simulink model "Q2_sim1"  (R2023b)
settings: Solver=VariableStepAuto  StartTime=0.0  StopTime=7  RelTol=1e-3
settings Model: Creator=avikd  LastModifiedBy=avikd

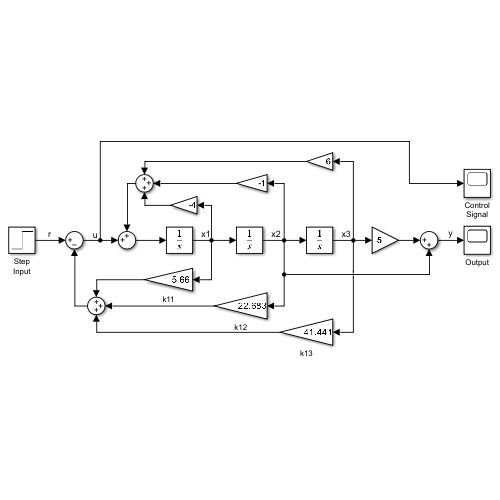
[thumbnail: Simulink's stored preview of the top-level diagram]
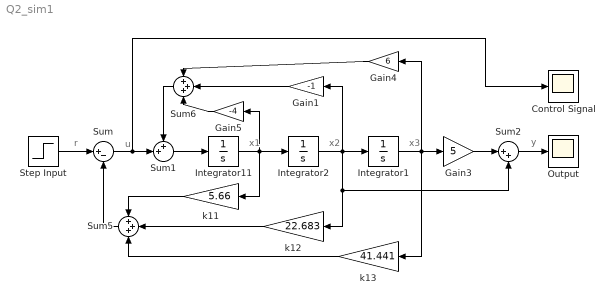
== system Q2_sim1 ==
  note: r
  note: u
  note: x3
  note: x2
  note: y
  note: x1
  Control Signal : Scope
  Gain1 : Gain  Gain=-1
  Gain3 : Gain  Gain=5
  Gain4 : Gain  Gain=6
  Gain5 : Gain  Gain=-4
  Integrator1 : Integrator
  Integrator11 : Integrator
  Integrator2 : Integrator
  Output : Scope
  Step Input : Step  Time=0  SampleTime=0
  Sum : Sum  Inputs=|+-
  Sum1 : Sum  Inputs=++|
  Sum2 : Sum  Inputs=|++
  Sum5 : Sum  Inputs=+++
  Sum6 : Sum  Inputs=+++
  k11 : Gain  Gain=5.66
  k12 : Gain  Gain=22.683
  k13 : Gain  Gain=41.441
  wires:
  Sum5/1 -> Sum/2
  Step Input/1 -> Sum/1
  Integrator11/1 -> k11/1, Integrator2/1, Gain5/1
  Integrator1/1 -> Gain4/1, k13/1, Gain3/1
  Gain3/1 -> Sum2/1
  Sum2/1 -> Output/1
  k11/1 -> Sum5/1
  k12/1 -> Sum5/2
  Sum/1 -> Control Signal/1, Sum1/2
  Sum6/1 -> Sum1/1
  Sum1/1 -> Integrator11/1
  k13/1 -> Sum5/3
  Integrator2/1 -> Gain1/1, Sum2/2, k12/1, Integrator1/1
  Gain5/1 -> Sum6/3
  Gain1/1 -> Sum6/2
  Gain4/1 -> Sum6/1
